simulink model "2021_03_30_Donghocthuan3DOF"  (R2018b)
settings: Solver=VariableStepAuto  StartTime=0.0  StopTime=10.0  RelTol=1e-3
settings Model: Creator=ADMIN  LastModifiedBy=ADMIN

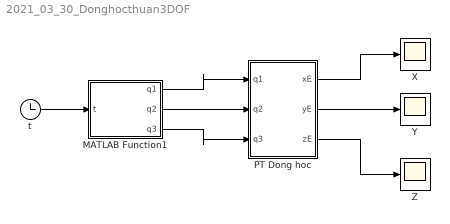
== system 2021_03_30_Donghocthuan3DOF ==
  MATLAB Function1 : MATLAB Function  TreatAsAtomicUnit=on
  PT Dong hoc : MATLAB Function  TreatAsAtomicUnit=on
  X : Scope
  Y : Scope
  Z : Scope
  t : Clock
  wires:
  PT Dong hoc/1(xE) -> X/1
  PT Dong hoc/2(yE) -> Y/1
  PT Dong hoc/3(zE) -> Z/1
  t/1 -> MATLAB Function1/1(t)
  MATLAB Function1/1(q1) -> PT Dong hoc/1(q1)
  MATLAB Function1/2(q2) -> PT Dong hoc/2(q2)
  MATLAB Function1/3(q3) -> PT Dong hoc/3(q3)

== matlab function 2021_03_30_Donghocthuan3DOF/MATLAB Function1 ==
  data: t input; q1 output; q2 output; q3 output
function [q1,q2,q3] = fcn(t)
q1=sin(t);
q2=cos(t);
q3=sin((pi/2)*t);

== matlab function 2021_03_30_Donghocthuan3DOF/PT Dong hoc ==
  data: q1 input; xE output; q2 input; q3 input; yE output; zE output
function [xE,yE,zE] = fcn(q1,q2,q3)
d1=100;
a2=60;
a3=40;

xE=cos(q1) * cos(q2) * a3 * cos(q3) - cos(q1) * sin(q2) * a3 * sin(q3) + cos(q1) * a2 * cos(q2);
yE=sin(q1) * cos(q2) * a3 * cos(q3) - sin(q1) * sin(q2) * a3 * sin(q3) + sin(q1) * a2 * cos(q2);
zE=sin(q2) * a3 * cos(q3) + cos(q2) * a3 * sin(q3) + a2 * sin(q2) + d1;
end
